simulink library "LiBatteryBlocks"  (R2019b)
settings: Solver=ode45  StartTime=0.0  StopTime=10.0  RelTol=1e-3  EnableMultiTasking=on
undefined symbols (not defined in the file): BatteryParams, numCells
libraries: fl_lib x13, $bdroot x8, LiBatteryElements_lib x4, nesl_utility x3, fl_ps_legacy_lib x1
settings Model: Creator=jgazzarr  LastModifiedBy=bhisma
settings DataIOCC: LimitDataPoints=on  SaveFormat=Array  SignalLoggingSaveFormat=ModelDataLogs  ReturnWorkspaceOutputs=off
settings OptimizationCC: ExpressionDepthLimit=2147483647  LifeSpan=inf
settings DebuggingCC: UnderspecifiedInitializationDetection=Classic  MergeDetectMultiDrivingBlocksExec=none  SolverPrmCheckMsg=warning  FcnCallInpInsideContextMsg=warning  StateNameClashWarn=warning  SFUnexpectedBacktrackingDiag=warning  SFNoUnconditionalDefaultTransitionDiag=warning  SFExecutionAtInitializationDiag=none  ArithmeticOperatorsInVariantConditions=warning
settings HardwareCC: ProdBitPerPointer=32  ProdBitPerSizeT=32  ProdBitPerPtrDiffT=32  ProdLargestAtomicFloat=None  ProdIntDivRoundTo=Undefined  ProdEndianess=Unspecified  ProdWordSize=32  ProdHWDeviceType=32-bit Generic
settings ModelReferenceCC: PropagateSignalLabelsOutOfModel=off
settings SFSimCC: SimUseLocalCustomCode=off  CustomCodeUndefinedFunction=UseInterfaceOnly
settings RTWCC: RTWUseLocalCustomCode=off
settings CodeAppCC: StateflowObjectComments=on
settings GRTTargetCC: TargetLangStandard=C89/C90 (ANSI)  GeneratePreprocessorConditionals=Disable all
settings ConfigComp: CovMetricSettings=dw  CovHtmlReporting=on  CovSaveCumulativeToWorkspaceVar=on  CovSaveSingleToWorkspaceVar=on  CovExternalEMLEnable=off

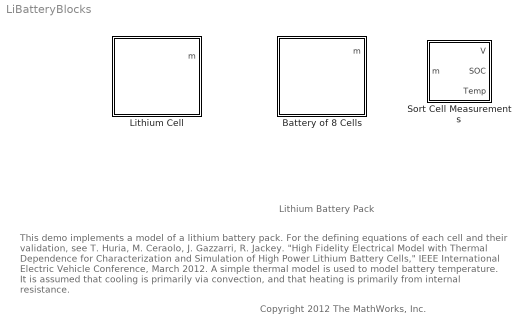
== system LiBatteryBlocks ==
  note: Lithium Battery Pack
  note: This demo implements a model of a lithium battery pack. For the defining equations of each cell and their validation, see T. Huria, M. Ceraolo,
      | J. Gazzarri, R. Jackey. "High Fidelity Electrical Model with Thermal Dependence for Characterization and Simulation of High Power Lithium
      | Battery Cells," IEEE International Electric Vehicle Conference, March 2012. A simple thermal model is used to model battery temperature. It is
      | assumed that cooling is primarily via convection, and that heating is primarily from internal resistance.
  note: Copyright 2012 The MathWorks, Inc.
  Battery of 8 Cells : Subsystem  mask(Battery 8 Series Cells){ThisStackParams=BatteryParams(1:8)}
      mask prompts: ThisStackParams "Parameter Structure (this stack of cells)"
      settings: AttributesFormatString=%<ThisStackParams>
  Lithium Cell : Subsystem  mask(Battery Cell){Battery=BatteryParams(1)}
      mask prompts: Battery "Battery Parameter Structure"
      settings: AttributesFormatString=%<Battery>
      mask Display:
      | image(imread('battery.jpg'))
      | color('red')
      | port_label('LConn',1,'+')
      | port_label('LConn',2,'-')
      | port_label('RConn',1,'H')
      | port_label('output',1,'m')
  Sort Cell Measurements : Subsystem

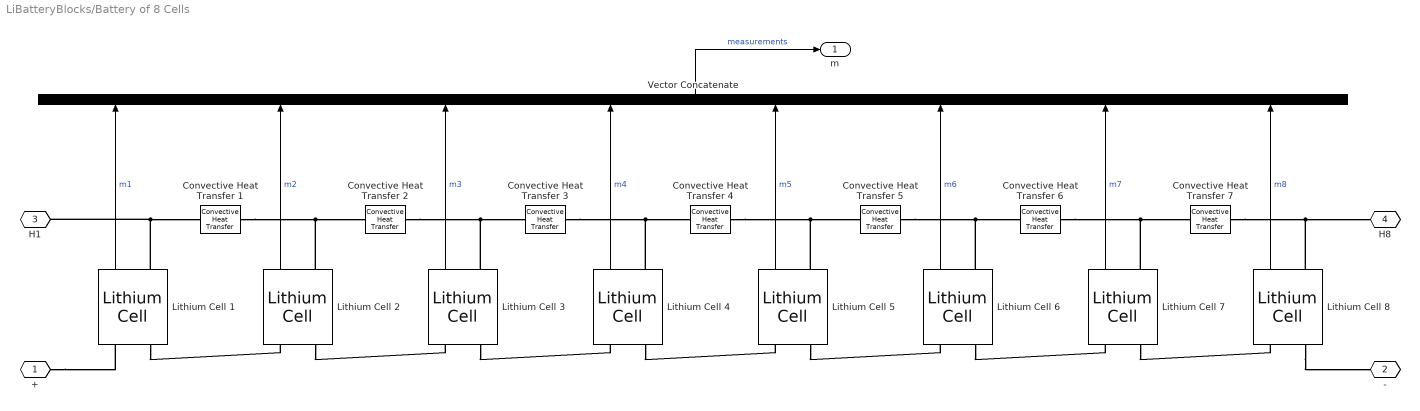
== system LiBatteryBlocks/Battery of 8 Cells ==
  Convective Heat Transfer {1..7} (7 alike) : fl_lib/Thermal/Thermal Elements/Convective Heat Transfer  area=cell_area m^2  heat_tr_coeff=h_conv W/(m^2 * K)  T_specify=off  T_priority=None  T=0 K  T_nominal_specify=off  T_nominal_unit=K  T_nominal_value=1  Q_specify=off  Q_priority=None  Q=0 W  Q_nominal_specify=off  Q_nominal_unit=W  Q_nominal_value=1
  Lithium Cell 1 : $bdroot/Lithium Cell  Battery=ThisStackParams(1)
      settings: AttributesFormatString=%<Battery>
  Lithium Cell 2 : $bdroot/Lithium Cell  Battery=ThisStackParams(2)
      settings: AttributesFormatString=%<Battery>
  Lithium Cell 3 : $bdroot/Lithium Cell  Battery=BatteryParams(3)
      settings: AttributesFormatString=%<Battery>
  Lithium Cell 4 : $bdroot/Lithium Cell  Battery=ThisStackParams(4)
      settings: AttributesFormatString=%<Battery>
  Lithium Cell 5 : $bdroot/Lithium Cell  Battery=ThisStackParams(5)
      settings: AttributesFormatString=%<Battery>
  Lithium Cell 6 : $bdroot/Lithium Cell  Battery=ThisStackParams(6)
      settings: AttributesFormatString=%<Battery>
  Lithium Cell 7 : $bdroot/Lithium Cell  Battery=ThisStackParams(7)
      settings: AttributesFormatString=%<Battery>
  Lithium Cell 8 : $bdroot/Lithium Cell  Battery=ThisStackParams(8)
      settings: AttributesFormatString=%<Battery>
  Vector Concatenate : Concatenate  NumInputs=8
  + : PMIOPort  Side=Left
  - : PMIOPort  Port=2  Side=Left
  H1 : PMIOPort  Port=3  Side=Right
  H8 : PMIOPort  Port=4  Side=Right
  m : Outport
  wires:
  Vector Concatenate/1 -> m/1  "measurements"
  Lithium Cell 8/1 -> Vector Concatenate/8  "m8"
  Lithium Cell 7/1 -> Vector Concatenate/7  "m7"
  Lithium Cell 6/1 -> Vector Concatenate/6  "m6"
  Lithium Cell 5/1 -> Vector Concatenate/5  "m5"
  Lithium Cell 4/1 -> Vector Concatenate/4  "m4"
  Lithium Cell 3/1 -> Vector Concatenate/3  "m3"
  Lithium Cell 2/1 -> Vector Concatenate/2  "m2"
  Lithium Cell 1/1 -> Vector Concatenate/1  "m1"
  connections:
  +/RConn1 -- Lithium Cell 1/LConn1
  Convective Heat Transfer 6/RConn1 -- Convective Heat Transfer 7/LConn1 -- Lithium Cell 7/RConn1
  Convective Heat Transfer 5/RConn1 -- Convective Heat Transfer 6/LConn1 -- Lithium Cell 6/RConn1
  Convective Heat Transfer 4/RConn1 -- Convective Heat Transfer 5/LConn1 -- Lithium Cell 5/RConn1
  Convective Heat Transfer 3/RConn1 -- Convective Heat Transfer 4/LConn1 -- Lithium Cell 4/RConn1
  Convective Heat Transfer 2/RConn1 -- Convective Heat Transfer 3/LConn1 -- Lithium Cell 3/RConn1
  Convective Heat Transfer 1/RConn1 -- Convective Heat Transfer 2/LConn1 -- Lithium Cell 2/RConn1
  Lithium Cell 8/LConn2 -- -/RConn1
  Lithium Cell 1/LConn2 -- Lithium Cell 2/LConn1
  Lithium Cell 2/LConn2 -- Lithium Cell 3/LConn1
  Lithium Cell 3/LConn2 -- Lithium Cell 4/LConn1
  Lithium Cell 4/LConn2 -- Lithium Cell 5/LConn1
  Lithium Cell 5/LConn2 -- Lithium Cell 6/LConn1
  Lithium Cell 6/LConn2 -- Lithium Cell 7/LConn1
  Lithium Cell 7/LConn2 -- Lithium Cell 8/LConn1
  Lithium Cell 1/RConn1 -- H1/RConn1 -- Convective Heat Transfer 1/LConn1
  Convective Heat Transfer 7/RConn1 -- H8/RConn1 -- Lithium Cell 8/RConn1

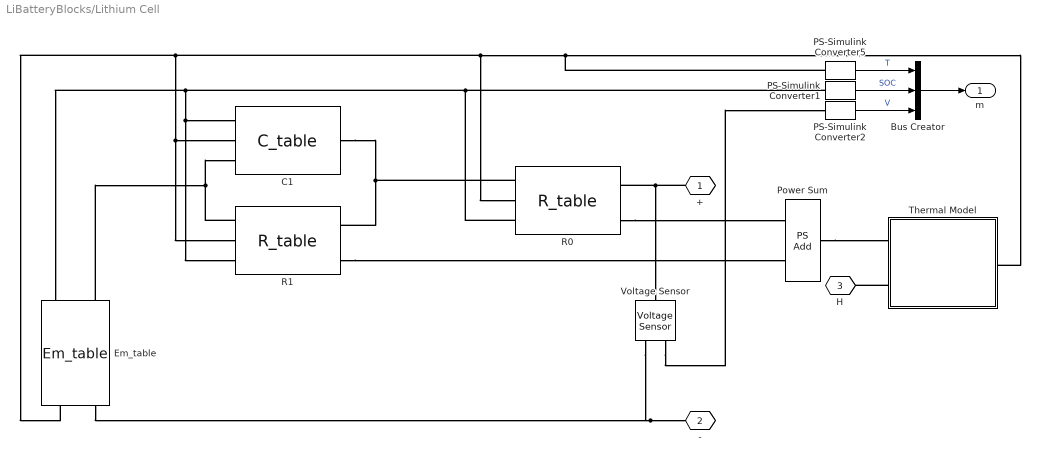
== system LiBatteryBlocks/Lithium Cell ==
  Bus Creator : BusCreator  Inputs=3
  C1 : LiBatteryElements_lib/C_table  C_Table=Battery.C1_LUT F  SOC_Table=Battery.SOC_LUT  Temp_Table=Battery.Temperature_LUT K  v0=0 V
      settings: InternalSimscapePortConfiguration="{\"Bottom\":[],\"Left\":[{\"id\":\"p\",\"label\":\"+\",\"type\":\"foundation.electrical.electrical\"},{\"id\":\"T\",\"label\":\"T\",\"type\":\"input\"},{\"id\":\"SOC\",\"label\":\"SOC\",\"type\":\"input\"}],\"Right\":[{\"id\":\"n\",\"label\":\"-\",\"type\":\"foundation.electrical.electrical\"}],\"Top\":[]}"
  Em_table : LiBatteryElements_lib/Em_table  C_Table=Battery.Capacity_LUT hr*A  Em_Table=Battery.Em_LUT V  SOC_Table=Battery.SOC_LUT  Temp_Table=Battery.Temperature_LUT K  Qinit=Battery.Qe_init hr*A
      settings: InternalSimscapePortConfiguration="{\"Bottom\":[],\"Left\":[{\"id\":\"p\",\"label\":\"+\",\"type\":\"foundation.electrical.electrical\"},{\"id\":\"C\",\"label\":\"C\",\"type\":\"output\"},{\"id\":\"SOC\",\"label\":\"SOC\",\"type\":\"output\"}],\"Right\":[{\"id\":\"n\",\"label\":\"-\",\"type\":\"foundation.electrical.electrical\"},{\"id\":\"T\",\"label\":\"T\",\"type\":\"input\"}],\"Top\":[]}"
  PS-Simulink Converter1 : nesl_utility/PS-Simulink Converter  PhysicalDomain=network_engine_domain  SubClassName=ps_output  LeftPortType=input  RightPortType=output  PseudoPeriodic=off  Frequencies=[]  Unit=1  AffineConversion=off
  PS-Simulink Converter2 : nesl_utility/PS-Simulink Converter  PhysicalDomain=network_engine_domain  SubClassName=ps_output  LeftPortType=input  RightPortType=output  PseudoPeriodic=off  Frequencies=[]  Unit=V  AffineConversion=off
  PS-Simulink Converter5 : nesl_utility/PS-Simulink Converter  PhysicalDomain=network_engine_domain  SubClassName=ps_output  LeftPortType=input  RightPortType=output  PseudoPeriodic=off  Frequencies=[]  Unit=C  AffineConversion=on
  Power Sum : fl_ps_legacy_lib/Legacy Physical Signals/Functions/PS Add
      settings: SourceProductName=Simscape  SourceProductBaseCode=SS  InternalSimscapePortConfiguration="{\"Bottom\":[],\"Left\":[{\"id\":\"I1\",\"label\":\"\",\"type\":\"input\"},{\"id\":\"I2\",\"label\":\"\",\"type\":\"input\"}],\"Right\":[{\"id\":\"O\",\"label\":\"\",\"type\":\"output\"}],\"Top\":[]}"
  R0 : LiBatteryElements_lib/R_table  R_Table=Battery.R0_LUT Ohm  SOC_Table=Battery.SOC_LUT  Temp_Table=Battery.Temperature_LUT K
      settings: InternalSimscapePortConfiguration="{\"Bottom\":[],\"Left\":[{\"id\":\"p\",\"label\":\"+\",\"type\":\"foundation.electrical.electrical\"},{\"id\":\"T\",\"label\":\"T\",\"type\":\"input\"},{\"id\":\"SOC\",\"label\":\"SOC\",\"type\":\"input\"}],\"Right\":[{\"id\":\"n\",\"label\":\"-\",\"type\":\"foundation.electrical.electrical\"},{\"id\":\"pow\",\"label\":\"POW\",\"type\":\"output\"}],\"Top\":[]}"
  R1 : LiBatteryElements_lib/R_table  R_Table=Battery.R1_LUT Ohm  SOC_Table=Battery.SOC_LUT  Temp_Table=Battery.Temperature_LUT K
      settings: InternalSimscapePortConfiguration="{\"Bottom\":[],\"Left\":[{\"id\":\"p\",\"label\":\"+\",\"type\":\"foundation.electrical.electrical\"},{\"id\":\"T\",\"label\":\"T\",\"type\":\"input\"},{\"id\":\"SOC\",\"label\":\"SOC\",\"type\":\"input\"}],\"Right\":[{\"id\":\"n\",\"label\":\"-\",\"type\":\"foundation.electrical.electrical\"},{\"id\":\"pow\",\"label\":\"POW\",\"type\":\"output\"}],\"Top\":[]}"
  Thermal Model : Subsystem
  Voltage Sensor : fl_lib/Electrical/Electrical Sensors/Voltage Sensor
  + : PMIOPort  Tag=PMCPort  Side=Left
  - : PMIOPort  Tag=PMCPort  Port=2  Side=Left
  H : PMIOPort  Tag=PMCPort  Port=3  Side=Right
  m : Outport
  wires:
  PS-Simulink Converter5/1 -> Bus Creator/1  "T"
  PS-Simulink Converter1/1 -> Bus Creator/2  "SOC"
  Bus Creator/1 -> m/1
  PS-Simulink Converter2/1 -> Bus Creator/3  "V"
  connections:
  R0/RConn2 -- Power Sum/LConn1
  R0/LConn1 -- C1/RConn1 -- R1/RConn1
  Power Sum/RConn1 -- Thermal Model/LConn1
  PS-Simulink Converter5/LConn1 -- C1/LConn2 -- R1/LConn2 -- Em_table/RConn2 -- R0/LConn2 -- Thermal Model/RConn1
  R1/RConn2 -- Power Sum/LConn2
  R1/LConn1 -- C1/LConn1 -- Em_table/LConn1
  +/RConn1 -- R0/RConn1 -- Voltage Sensor/LConn1
  Em_table/RConn1 -- -/RConn1 -- Voltage Sensor/RConn2
  Thermal Model/LConn2 -- H/RConn1
  PS-Simulink Converter1/LConn1 -- C1/LConn3 -- R1/LConn3 -- Em_table/LConn3 -- R0/LConn3
  Voltage Sensor/RConn1 -- PS-Simulink Converter2/LConn1

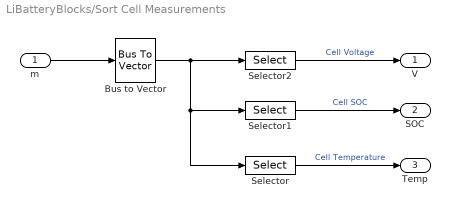
== system LiBatteryBlocks/Sort Cell Measurements ==
  m : Inport
  Bus to Vector : BusToVector
  Selector : Selector  InputPortWidth=numCells * 3  IndexOptions=Index vector (dialog)  Indices=1:3:numCells*3  OutputSizes=1
  Selector1 : Selector  InputPortWidth=numCells * 3  IndexOptions=Index vector (dialog)  Indices=2:3:numCells*3  OutputSizes=1
  Selector2 : Selector  InputPortWidth=numCells * 3  IndexOptions=Index vector (dialog)  Indices=3:3:numCells*3  OutputSizes=1
  V : Outport
  SOC : Outport  Port=2
  Temp : Outport  Port=3
  wires:
  Selector2/1 -> V/1  "Cell Voltage"
  Selector1/1 -> SOC/1  "Cell SOC"
  Selector/1 -> Temp/1  "Cell Temperature"
  Bus to Vector/1 -> Selector1/1, Selector/1, Selector2/1
  m/1 -> Bus to Vector/1

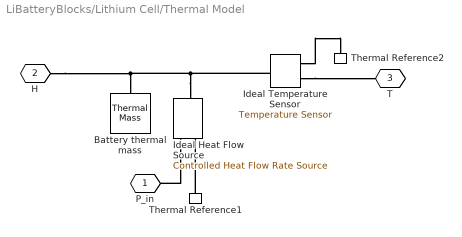
== system LiBatteryBlocks/Lithium Cell/Thermal Model ==
  Battery thermal mass : fl_lib/Thermal/Thermal Elements/Thermal Mass  mass=Battery.cell_mass kg  sp_heat=Battery.cell_Cp_heat J/kg/K  T_specify=on  T_priority=High  T=Battery.T_init K  T_nominal_specify=off  T_nominal_unit=K  T_nominal_value=1  Q_specify=off  Q_priority=None  Q=0 W  Q_nominal_specify=off  Q_nominal_unit=W  Q_nominal_value=1
  Ideal Temperature Sensor : fl_lib/Thermal/Thermal Sensors/Temperature Sensor
  Ideal Heat Flow Source : fl_lib/Thermal/Thermal Sources/Controlled Heat Flow Rate Source
      settings: SourceProductName=Simscape
  Thermal Reference1 : fl_lib/Thermal/Thermal Elements/Thermal Reference
  Thermal Reference2 : fl_lib/Thermal/Thermal Elements/Thermal Reference
  P_in : PMIOPort  Tag=PMCPort  Side=Left
  H : PMIOPort  Tag=PMCPort  Port=2  Side=Left
  T : PMIOPort  Tag=PMCPort  Port=3  Side=Right
  connections:
  Ideal Heat Flow Source/RConn1 -- P_in/RConn1
  Ideal Heat Flow Source/LConn1 -- Battery thermal mass/LConn1 -- H/RConn1 -- Ideal Temperature Sensor/LConn1
  Thermal Reference1/LConn1 -- Ideal Heat Flow Source/RConn2
  Ideal Temperature Sensor/RConn2 -- T/RConn1
  Ideal Temperature Sensor/RConn1 -- Thermal Reference2/LConn1
